simulink model "absbrake"  (Simulink 6.0)
settings: Solver=ode45  SolverMode=SingleTasking  StartTime=0.0  StopTime=25  MaxStep=.01  RelTol=1e-3  AbsTol=1e-6
PreLoadFcn:
  | absdata
values from neighbouring files (symbols this model uses):
  ctrl = 1    [absdata.m]
  g = 32.18    [absdata.m]
  I = 5    [absdata.m]
  Kf = 1    [absdata.m]
  m = 50    [absdata.m]
  mu = [0 .4 .8 .97 1.0 .98 .96 .94 .92 .9 .88 .855 .83 .81 .79 .77 .75 .73 .72 .71 .7]    [absdata.m]
  PBmax = 1500    [absdata.m]
  Rr = 15/12    (= 1.25)    [absdata.m]
  slip = (0:.05:1.0)    [absdata.m]
  TB = 0.01    [absdata.m]
  v0 = 88    [absdata.m]
settings Model: Creator=The MathWorks Inc.  LastModifiedBy=batserve  ExtModeTrigMode=oneshot  ExtModeArmWhenConnect=off  ExtModeAutoUpdateStatusClock=off
settings DataIOCC: LimitDataPoints=off  SaveOutput=off  TimeSaveName=time
settings DebuggingCC: CheckExecutionContextPreStartOutputMsg=on  CheckExecutionContextRuntimeOutputMsg=on  SolverPrmCheckMsg=none  IntegerOverflowMsg=none
settings HardwareCC: TargetUnknown=on

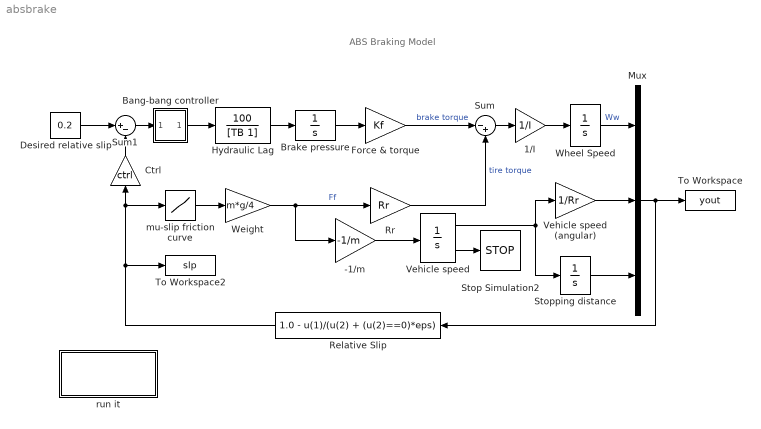
== system absbrake ==
  note: ABS Braking Model
  -1/m : Gain  Gain=-1/m  SaturateOnIntegerOverflow=on
  1/I : Gain  Gain=1/I  SaturateOnIntegerOverflow=on
  Bang-bang controller : Subsystem  PropExecContextAcrossSSBoundary=on
      mask Type: Sign
      mask Description: y = sign(x)
      mask Help: Sign Function:\n\t\t\ty = 1 if x > 0\n\t\t\ty = 0 if x = 0\n\t\t\ty = -1 if x < 0
      mask Display: plot(-50,-50,50,50,[-50,50],[0,0],[0,0],[-50,50],[-40,0],[-30,-30],[0,40],[30,30])
  Brake pressure : Integrator  LimitOutput=on  UpperSaturationLimit=PBmax  LowerSaturationLimit=0
  Ctrl : Gain  Orientation=up  Gain=ctrl  SaturateOnIntegerOverflow=on
  Desired relative slip : Constant  Value=0.2
  Force & torque : Gain  Gain=Kf  SaturateOnIntegerOverflow=on
  "Hydraulic Lag " : TransferFcn  Numerator=[100]  Denominator=[TB 1]
  Mux : Mux  Inputs=3
  Relative Slip : Fcn  Orientation=left  Expr=1.0 - u(1)/(u(2) + (u(2)==0)*eps)
  Rr : Gain  Gain=Rr  SaturateOnIntegerOverflow=on
  Stop Simulation2 : Stop
  Stopping distance : Integrator  UpperSaturationLimit=1000  LowerSaturationLimit=0
  Sum : Sum  Inputs=|-+  SaturateOnIntegerOverflow=on  InputSameDT=on
  Sum1 : Sum  Inputs=|+-  SaturateOnIntegerOverflow=on  InputSameDT=on
  To Workspace : ToWorkspace  VariableName=yout  SaveFormat=Array
      settings: MaxDataPoints=10000
  To Workspace2 : ToWorkspace  VariableName=slp  SaveFormat=Array
      settings: MaxDataPoints=10000
  Vehicle speed : Integrator  InitialCondition=v0  LimitOutput=on  UpperSaturationLimit=1000  LowerSaturationLimit=0  ShowSaturationPort=on
  Vehicle speed (angular) : Gain  Gain=1/Rr  SaturateOnIntegerOverflow=on
  Weight : Gain  Gain=m*g/4  SaturateOnIntegerOverflow=on
  Wheel Speed : Integrator  InitialCondition=v0/Rr  LimitOutput=on  UpperSaturationLimit=1000  LowerSaturationLimit=0
  mu-slip friction curve : Lookup  DialogController=Simulink.DDGSource  InputValues=slip  OutputValues=mu  SaturateOnIntegerOverflow=on
  run it : Subsystem  PropExecContextAcrossSSBoundary=on
      settings: OpenFcn=runabs
      mask Display: disp('Double click to\nrun model and\nplot the results')
  wires:
  1/I/1 -> Wheel Speed/1
  Mux/1 -> To Workspace/1, Relative Slip/1
  Sum/1 -> 1/I/1
  Wheel Speed/1 -> Mux/1  "Ww"
  Vehicle speed (angular)/1 -> Mux/2
  Relative Slip/1 -> To Workspace2/1, mu-slip friction curve/1, Ctrl/1
  Rr/1 -> Sum/2  "tire torque"
  Force & torque/1 -> Sum/1  "brake torque"
  Stopping distance/1 -> Mux/3
  -1/m/1 -> Vehicle speed/1
  Vehicle speed/2 -> Stop Simulation2/1
  Vehicle speed/1 -> Vehicle speed (angular)/1, Stopping distance/1
  mu-slip friction curve/1 -> Weight/1
  Weight/1 -> -1/m/1, Rr/1  "Ff"
  Brake pressure/1 -> Force & torque/1
  Ctrl/1 -> Sum1/2
  Bang-bang controller/1(out_1) -> "Hydraulic Lag "/1
  "Hydraulic Lag "/1 -> Brake pressure/1
  Desired relative slip/1 -> Sum1/1
  Sum1/1 -> Bang-bang controller/1(in_1)

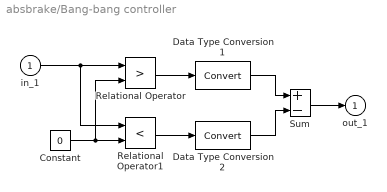
== system absbrake/Bang-bang controller ==
  in_1 : Inport  Port=1  LatchInput=off
  Constant : Constant  Value=0
  Data Type Conversion1 : DataTypeConversion  OutDataTypeMode=double  SaturateOnIntegerOverflow=on  RndMeth=Zero
  Data Type Conversion2 : DataTypeConversion  OutDataTypeMode=double  SaturateOnIntegerOverflow=on  RndMeth=Zero
  Relational Operator : RelationalOperator  Operator=>  InputSameDT=on
  Relational Operator1 : RelationalOperator  Operator=<  InputSameDT=on
  Sum : Sum  Inputs=+-  SaturateOnIntegerOverflow=on  InputSameDT=on
  out_1 : Outport  InitialOutput=0
  wires:
  in_1/1 -> Relational Operator/1, Relational Operator1/1
  Constant/1 -> Relational Operator1/2, Relational Operator/2
  Relational Operator1/1 -> Data Type Conversion2/1
  Relational Operator/1 -> Data Type Conversion1/1
  Sum/1 -> out_1/1
  Data Type Conversion1/1 -> Sum/1
  Data Type Conversion2/1 -> Sum/2

== system absbrake/run it ==
